simulink model "TestPDUCDULUTAssembly"  (R2025b)
settings: Solver=daessc  StartTime=0.0  StopTime=1200  MaxStep=1  RelTol=1e-3  AbsTol=1e-3
libraries: nesl_utility x7, fl_lib x6, datacenterCompositeLib x1
settings Model: Creator=vikrants  LastModifiedBy=vikrants
settings SolverCC: AutoScaleAbsTol=off  AlgebraicLoopSolver=TrustRegion  MaxZcPerStep=1.0
settings DebuggingCC: UnconnectedInputMsg=warning  UnconnectedOutputMsg=warning  UnconnectedLineMsg=warning  SymbolicDimsDataTypeCodeGenerationDiagnostic=none
settings ModelReferenceCC: EnableRefExpFcnMdlSchedulingChecks=on
settings SFSimCC: CustomCodeUndefinedFunction=UseInterfaceOnly
settings RTWCC: GPUComputeCapability=3.5  DLArmComputeVersion=19.05
settings SimscapeCC: SimscapeLogType=all  SimscapeLogSimulationStatistics=on  SimscapeLogDataHistory=10000.0

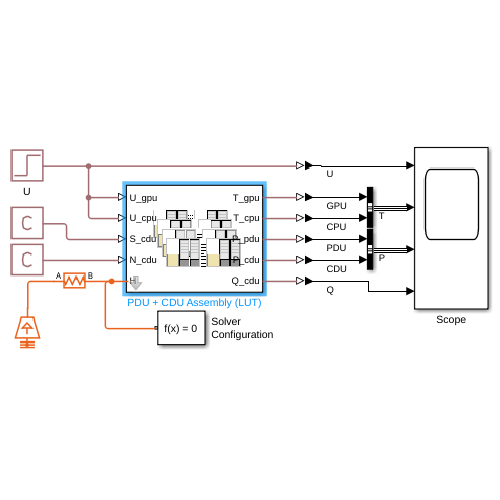
[thumbnail: Simulink's stored preview of the top-level diagram]
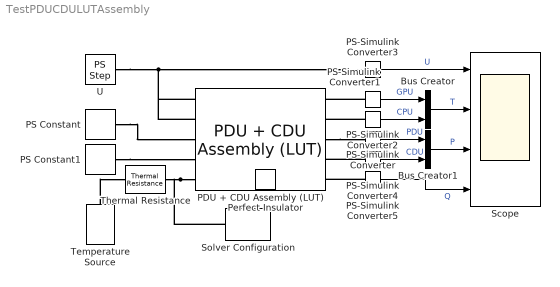
== system TestPDUCDULUTAssembly ==
  Bus Creator : BusCreator  Inputs=2
  Bus Creator1 : BusCreator  Inputs=2
  PDU + CDU Assembly (LUT) : datacenterCompositeLib/PDU + CDU Assembly (LUT)  nAssembly=3  nRacks=4  nTrays=6  flowrate_vec=[0.1:0.1:1]/998  capacity_vec=50000*ones(1,10)  numPump=2  effPump_vec=[0.4,0.42,0.45,0.5,0.55,0.6,0.62,0.65,0.65,0.64]  prDrop_mat=1000*[0.28,1.11,2.5,4.44,6.94,10,13.61,17.78,22.5,27.78; 5.6,2.22,5,8.88,13.88,20,27.22,35.56,45,55.56]'  speed=1  trayMass=5  trayCp=2000  trayThermalR=0.1  nGPU=1  gpuTDPperDie=1200  gpuIdlePower=300  gpuHBMpower=80  gpuExponent=1.4  gpuHBMutil=0.7  gpuLeakage=1.5  gpuNominalDieT=350  gpuDieThermalC=50  gpuHeatSinkR=0.15  gpuSurfArea=0.01  gpuAmbientR=0.5  nCPU=1  cpuTDPperSocket=350  cpuIdlePower=80  cpuExponent=1.1  cpuLeakage=1.5  cpuNominalDieT=350  cpuDieThermalC=50  cpuHeatSinkR=0.15  cpuSurfArea=0.01  cpuAmbientR=0.5  initialT=350  htc=10
  PS Constant : fl_lib/Physical Signals/Sources/PS Constant  constant=1
  PS Constant1 : fl_lib/Physical Signals/Sources/PS Constant  constant=1
  PS-Simulink Converter{,1..5} (6 alike) : nesl_utility/PS-Simulink Converter  PhysicalDomain=network_engine_domain  SubClassName=ps_output  LeftPortType=input  RightPortType=output  PseudoPeriodic=off  Frequencies=[]  VectorFormat=inherit  Unit=inherit  AffineConversion=off
  Perfect Insulator : fl_lib/Thermal/Thermal Elements/Perfect Insulator  T_specify=off  T_priority=None  T=293.15 K  T_nominal_specify=off  T_nominal_value=1  T_nominal_unit=K
  Scope : Scope  NumInputPorts=4
      settings: ActiveDisplayYMinimum=0.15000000000000002  ActiveDisplayYMaximum=0.64999999999999991
  Solver Configuration : nesl_utility/Solver Configuration  PhysicalDomain=network_engine_domain  SubClassName=solver  LeftPortType=input  RightPortType=generic  Tones=[]  Harmonics=[]  SimulateNoise=off  Profile=off  UseLocalSampling=off  EnableSwitchedLinearOptims=on  FrequencyDomain=off  UseCCode=off  RelTol=0.001  AbsTol=1e-06  MinStep=1e-09  ToWorkspace=off  RevertToSquareIcSolve=off  NumHomotopyIterations=100  PhasorMode=off  PhasorModeNumHarmonics=1  ConsistencySolver=NEWTON_XTOL_AFTER_FTOL  IndexReductionMethod=DerivativeReplacement  DoDC=off  ResidualTolerance=1e-09  ConsistencyTolSource=GLOBAL  ConsistencyAbsTol=0.001  ConsistencyRelTol=0.001  ConsistencyTolFactor=0.001  UseLocalSolver=off  LocalSolverChoice=NE_BACKWARD_EULER_ADVANCER  ResolveIndetEquations=on  FunctionEvalNumThread=1  LocalSolverSampleTime=0.001  DoFixedCost=off  MaxNonlinIter=3  MaxModeIter=2  ComputeImpulses=off  ImpulseIterations=2  LinearAlgebra=auto  LinearAlgebraNumThread=0  EquationFormulation=NE_TIME_EF  DelaysMemoryBudget=1024  AutomaticFiltering=on  FilteringTimeConstant=0.001  PartitionStorageMethod=AS_NEEDED  PartitionMemoryBudget=1024  PartitionMethod=ROBUST  MultibodyUseLocalSolver=off  MultibodyLocalSolverChoice=ODE1  MultibodyLocalSolverSampleTime=0.001
  Temperature Source : fl_lib/Thermal/Thermal Sources/Temperature Source  temperature=293.15 K
  Thermal Resistance : fl_lib/Thermal/Thermal Elements/Thermal Resistance  resistance=1e-2 K/W  T_specify=off  T_priority=None  T=0 K  T_nominal_specify=off  T_nominal_value=1  T_nominal_unit=K  Q_specify=off  Q_priority=None  Q=0 W  Q_nominal_specify=off  Q_nominal_value=1  Q_nominal_unit=W
  U : fl_lib/Physical Signals/Sources/PS Step  step_time=600 s  initial_value=0.6  final_value=0.2
  wires:
  PS-Simulink Converter1/1 -> Bus Creator/1  "GPU"
  PS-Simulink Converter2/1 -> Bus Creator/2  "CPU"
  PS-Simulink Converter3/1 -> Scope/1  "U"
  PS-Simulink Converter/1 -> Bus Creator1/1  "PDU"
  PS-Simulink Converter4/1 -> Bus Creator1/2  "CDU"
  Bus Creator/1 -> Scope/2  "T"
  Bus Creator1/1 -> Scope/3  "P"
  PS-Simulink Converter5/1 -> Scope/4  "Q"
  connections:
  U/RConn1 -- PDU + CDU Assembly (LUT)/LConn2 -- PDU + CDU Assembly (LUT)/LConn1 -- PS-Simulink Converter3/LConn1
  Thermal Resistance/RConn1 -- Solver Configuration/RConn1 -- PDU + CDU Assembly (LUT)/LConn5
  Temperature Source/LConn1 -- Thermal Resistance/LConn1
  PS-Simulink Converter2/LConn1 -- PDU + CDU Assembly (LUT)/RConn2
  PS-Simulink Converter1/LConn1 -- PDU + CDU Assembly (LUT)/RConn1
  PS-Simulink Converter4/LConn1 -- PDU + CDU Assembly (LUT)/RConn4
  PDU + CDU Assembly (LUT)/RConn3 -- PS-Simulink Converter/LConn1
  PS-Simulink Converter5/LConn1 -- PDU + CDU Assembly (LUT)/RConn5
  PS Constant/RConn1 -- PDU + CDU Assembly (LUT)/LConn3
  PS Constant1/RConn1 -- PDU + CDU Assembly (LUT)/LConn4
